simulink model "question49"  (R2024a)
settings: Solver=VariableStepAuto  StartTime=0.0  StopTime=10.0  RelTol=1e-3
settings Model: Creator=roboticslab  LastModifiedBy=roboticslab

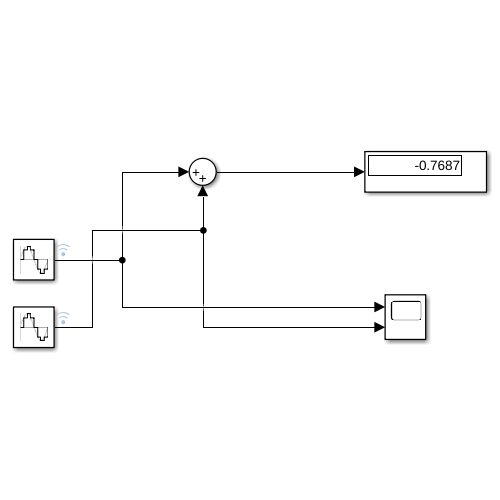
[thumbnail: Simulink's stored preview of the top-level diagram]
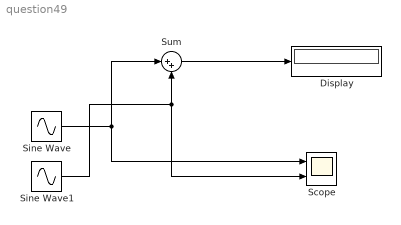
== system question49 ==
  Display : Display
  Scope : Scope  NumInputPorts=2
  Sine Wave : Sin  Frequency=5  SampleTime=1
  Sine Wave1 : Sin  Frequency=10  SampleTime=1
  Sum : Sum  Inputs=|++
  wires:
  Sine Wave/1 -> Scope/1, Sum/1
  Sum/1 -> Display/1
  Sine Wave1/1 -> Scope/2, Sum/2
